simulink model "EngReq"  (R2018a)
settings: configuration reference "cs_ert" (kept outside this file)
settings Model: DataDictionary=EngReq.sldd  Creator=zhoutinglin  LastModifiedBy=zhoutinglin

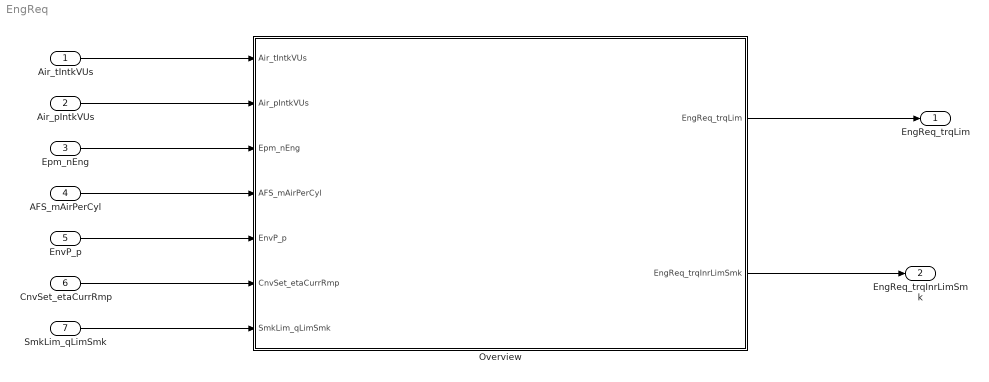
== system EngReq ==
  Air_tIntkVUs : Inport
  Air_pIntkVUs : Inport  Port=2
  Epm_nEng : Inport  Port=3
  AFS_mAirPerCyl : Inport  Port=4
  EnvP_p : Inport  Port=5
  CnvSet_etaCurrRmp : Inport  Port=6
  SmkLim_qLimSmk : Inport  Port=7
  Overview : Subsystem
  EngReq_trqLim : Outport
  EngReq_trqInrLimSmk : Outport  Port=2
  wires:
  Air_tIntkVUs/1 -> Overview/1(Air_tIntkVUs)
  Air_pIntkVUs/1 -> Overview/2(Air_pIntkVUs)
  Epm_nEng/1 -> Overview/3(Epm_nEng)
  AFS_mAirPerCyl/1 -> Overview/4(AFS_mAirPerCyl)
  EnvP_p/1 -> Overview/5(EnvP_p)
  CnvSet_etaCurrRmp/1 -> Overview/6(CnvSet_etaCurrRmp)
  SmkLim_qLimSmk/1 -> Overview/7(SmkLim_qLimSmk)
  Overview/1(EngReq_trqLim) -> EngReq_trqLim/1
  Overview/2(EngReq_trqInrLimSmk) -> EngReq_trqInrLimSmk/1

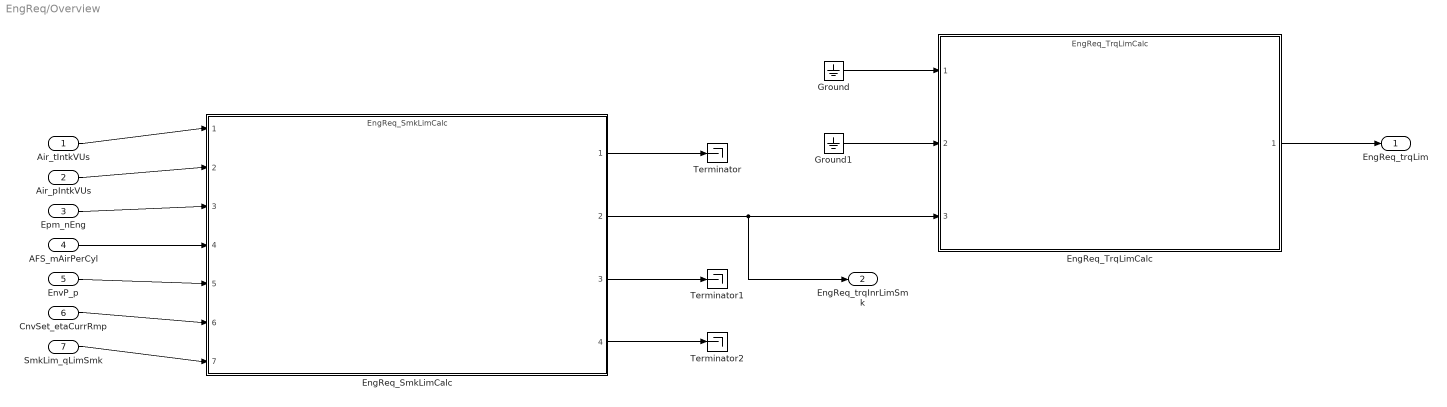
== system EngReq/Overview ==
  Air_tIntkVUs : Inport
  Air_pIntkVUs : Inport  Port=2
  Epm_nEng : Inport  Port=3
  AFS_mAirPerCyl : Inport  Port=4
  EnvP_p : Inport  Port=5
  CnvSet_etaCurrRmp : Inport  Port=6
  SmkLim_qLimSmk : Inport  Port=7
  EngReq_SmkLimCalc : ModelReference  ModelNameDialog=EngReq_SmkLimCalc  SimulationMode=Normal  ModelReferenceVersion=1.51
  EngReq_TrqLimCalc : ModelReference  ModelNameDialog=EngReq_TrqLimCalc  SimulationMode=Normal  ModelReferenceVersion=1.49
  Ground : Ground
  Ground1 : Ground
  Terminator : Terminator
  Terminator1 : Terminator
  Terminator2 : Terminator
  EngReq_trqLim : Outport
  EngReq_trqInrLimSmk : Outport  Port=2
  wires:
  EngReq_SmkLimCalc/2 -> EngReq_trqInrLimSmk/1, EngReq_TrqLimCalc/3
  Air_tIntkVUs/1 -> EngReq_SmkLimCalc/1
  Air_pIntkVUs/1 -> EngReq_SmkLimCalc/2
  Epm_nEng/1 -> EngReq_SmkLimCalc/3
  AFS_mAirPerCyl/1 -> EngReq_SmkLimCalc/4
  EnvP_p/1 -> EngReq_SmkLimCalc/5
  CnvSet_etaCurrRmp/1 -> EngReq_SmkLimCalc/6
  SmkLim_qLimSmk/1 -> EngReq_SmkLimCalc/7
  EngReq_SmkLimCalc/1 -> Terminator/1
  EngReq_SmkLimCalc/3 -> Terminator1/1
  EngReq_SmkLimCalc/4 -> Terminator2/1
  EngReq_TrqLimCalc/1 -> EngReq_trqLim/1
  Ground/1 -> EngReq_TrqLimCalc/1
  Ground1/1 -> EngReq_TrqLimCalc/2
